simulink model "Modell_PID"  (R2023a)
settings: Solver=VariableStepAuto  StartTime=0.0  StopTime=480  FixedStep=1/30  RelTol=1e-3
undefined symbols (not defined in the file or in its folder): DiscIntNeverNeededParam, dsys, gray, LF, none, videoinput
libraries: instrumentseriallib x3, visiontextngfix x2, slident x2, svdutilitieslib x1, imaqlib x1, simulink_extras x1, simulink x1
settings Model: Creator=Legenden-PC  LastModifiedBy=Legenden-PC
settings OptimizationCC: ReuseModelBlockBuffer=off

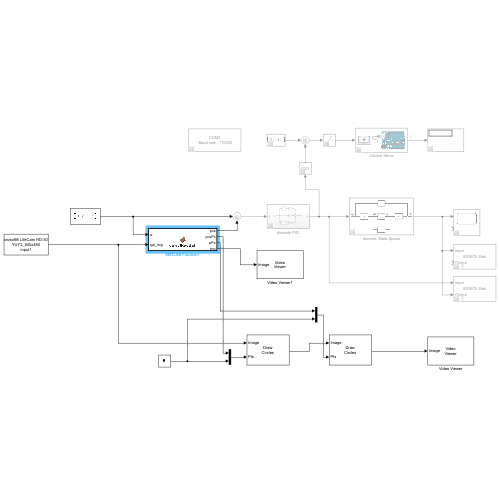
[thumbnail: Simulink's stored preview of the top-level diagram]
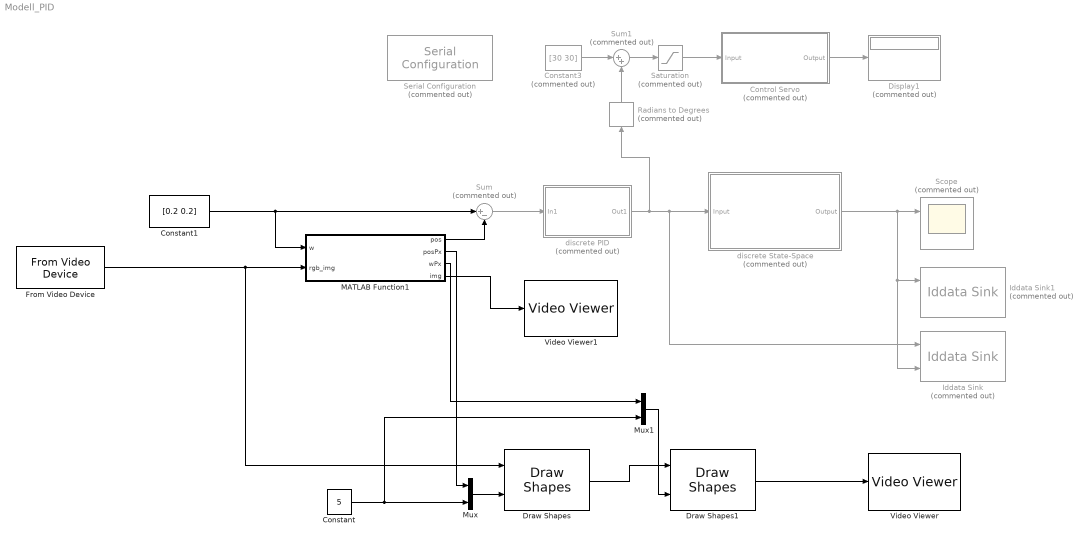
== system Modell_PID ==
  Constant : Constant  Value=5  VectorParams1D=off
  Constant1 : Constant  Value=[0.2 0.2]  SampleTime=1/30
  Constant3 : Constant  Commented=on  Value=[30 30]
  Control Servo : Subsystem  Commented=on
      mask Display: image('C:\Users\Legenden-PC\Desktop\arduino_usb.png'); % Use "Edit Image" on toolstrip to change.
  Display1 : Display  Commented=on
  Draw Shapes : visiontextngfix/Draw Shapes  shape=Circles  fill=off  lineWidth=3  fillClrSource=Specify via dialog  display=Black  intensity=200  color=[200 255 100]  opacity=0.6  viewport=Entire image  antialiasing=off  inType=Obsolete  imagePorts=One multidimensional signal  roundingMode=Floor  overflowMode=off  memoryMode=Specify word length  memoryWordLength=16  prodOutputMode=Binary point scaling  prodOutputWordLength=32  prodOutputFracLength=14  memoryFracLength=15
  Draw Shapes1 : visiontextngfix/Draw Shapes  shape=Circles  fill=off  lineWidth=3  fillClrSource=Specify via dialog  display=Black  intensity=200  color=[200 255 100]  opacity=0.6  viewport=Entire image  antialiasing=off  inType=Obsolete  imagePorts=One multidimensional signal  roundingMode=Floor  overflowMode=off  memoryMode=Specify word length  memoryWordLength=16  prodOutputMode=Binary point scaling  prodOutputWordLength=32  prodOutputFracLength=14  memoryFracLength=15
  From Video Device : imaqlib/From Video Device  DeviceMenu=winvideo 2 (Microsoft® LifeCam HD-3000)  Device=winvideo 2 (Microsoft® LifeCam HD-3000)  ObjConstructor=videoinput('winvideo', 2)  VideoFormatMenu=YUY2_640x480  VideoFormat=YUY2_640x480  VideoSource=input1  ROIPosition=[0 60 480 480]  EnableHWTrigger=off  TriggerConfiguration=none/none  SampleTime=1/30  OutputPortsMode=One multidimensional signal  DataType=single  CanDoHWTrigger=no  ReturnedColorSpace=rgb  BlockHandle=10250.0001  ROIWidth=480  ROIHeight=480  ROIColumn=60  ROIRow=0  EngXMLPath=C:\Program Files\MATLAB\R2023a\toolbox\imaq\imaq\private  DevXMLPath=C:\ProgramData\MATLAB\SupportPackages\R2023a\toolbox\imaq\supportpackages\genericvideo\adaptor\win64  EngLibPath=C:\Program Files\MATLAB\R2023a\toolbox\imaq\imaqblks\imaqmex\win64  ColorSpace=rgb  BayerSensorAlignment=grbg  ImaqMode=off
  Iddata Sink : slident/Iddata Sink  Commented=on  datasetname=ymodel  Ts=1/30  isu=off  isy=off
  Iddata Sink1 : slident/Iddata Sink  Commented=on  datasetname=w_vs_model  Ts=1/30  isu=off  isy=off
  MATLAB Function1 : MATLAB Function  TreatAsAtomicUnit=on
  Mux : Mux  Inputs=2
  Mux1 : Mux  Inputs=2
  Radians to Degrees : simulink_extras/Transformations/Radians to Degrees  Commented=on
  Saturation : Saturate  Commented=on  UpperLimit=60  LowerLimit=0
  Scope : Scope  Commented=on  NumInputPorts=2
  Serial Configuration : instrumentseriallib/Serial Configuration  Priority=-200000  Commented=on  PortSel=COM3  Port=COM3  ComPort=COM3  BaudRate=115200  DataBits=8  Parity=none  StopBits=1  ByteOrder=little-endian  FlowControl=none  Timeout=10  SimulateUsing=Interpreted execution  BlockInModel=on  aMode=1
  Sum : Sum  Commented=on  Inputs=|+-
  Sum1 : Sum  Commented=on  Inputs=|++
  Video Viewer : VideoViewer  colormapValue=gray(256)  FigPos=[1 1030 1920 930]
  Video Viewer1 : VideoViewer  FigPos=[470 761 614 489]
  discrete PID : Subsystem  Commented=on
  discrete State-Space : Subsystem  Commented=on
      mask Display: image('$imagefile'); % Use "Edit Image" on toolstrip to change.
  wires:
  discrete State-Space/1(Output) -> Iddata Sink1/1, Iddata Sink/2, Scope/1
  Sum/1 -> discrete PID/1(In1)
  discrete PID/1(Out1) -> Iddata Sink/1, discrete State-Space/1(Input), Radians to Degrees/1
  From Video Device/1 -> Draw Shapes/1, MATLAB Function1/2(rgb_img)
  Mux/1 -> Draw Shapes/2
  Constant/1 -> Mux1/2, Mux/2
  MATLAB Function1/2(posPx) -> Mux/1
  MATLAB Function1/1(pos) -> Sum/2
  Saturation/1 -> Control Servo/1(Input)
  Sum1/1 -> Saturation/1
  Control Servo/1(Output) -> Display1/1
  Radians to Degrees/1 -> Sum1/2
  Constant3/1 -> Sum1/1
  Draw Shapes/1 -> Draw Shapes1/1
  Draw Shapes1/1 -> Video Viewer/1
  Mux1/1 -> Draw Shapes1/2
  MATLAB Function1/3(wPx) -> Mux1/1
  Constant1/1 -> Sum/1, MATLAB Function1/1(w)
  MATLAB Function1/4(img) -> Video Viewer1/1

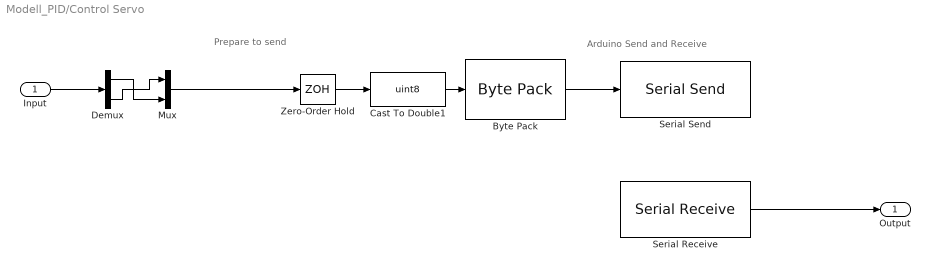
== system Modell_PID/Control Servo ==
  note: Prepare to send
  note: Arduino Send and Receive
  Input : Inport
  Byte Pack : svdutilitieslib/Byte Pack  maskPackedDataType=uint8  datatypes={'uint8'}  byteAlign=2  blockPlatform=arduinoert
  Cast To Double1 : DataTypeConversion  OutDataTypeStr=uint8  SaturateOnIntegerOverflow=off  RndMeth=Floor
  Demux : Demux  Outputs=2
  Mux : Mux  Inputs=2
  Serial Receive : instrumentseriallib/Serial Receive  PortSel=COM3  Port=COM3  ComPort=COM3  DataType=uint8  SaveDataType=uint8  ToggleHeader=on  Header=[ 65 ]  ToggleTerminator=on  Terminator=LF ('\n')  CustomTerminator=[]  InputFormat=Column major  ToggleDataSize=on  DataSize="[1  2]"  EnableBlockingMode=on  ActionDataUnavailable=Output last received value  ActionWhenDataUnavailable=Output last received value  CustomValue=0  SampleTime=0.01  SimulateUsing=Interpreted execution  BlockInModel=on  aMode=1
  Serial Send : instrumentseriallib/Serial Send  PortSel=COM3  Port=COM3  ComPort=COM3  Header=[]  Terminator=<none>  CustomTerminator=[]  EnableBlockingMode=on  SimulateUsing=Interpreted execution  BlockInModel=on  aMode=1
  Zero-Order Hold : ZeroOrderHold  SampleTime=0.01
  Output : Outport
  wires:
  Cast To Double1/1 -> Byte Pack/1
  Byte Pack/1 -> Serial Send/1
  Serial Receive/1 -> Output/1
  Zero-Order Hold/1 -> Cast To Double1/1
  Input/1 -> Demux/1
  Demux/1 -> Mux/2
  Demux/2 -> Mux/1
  Mux/1 -> Zero-Order Hold/1

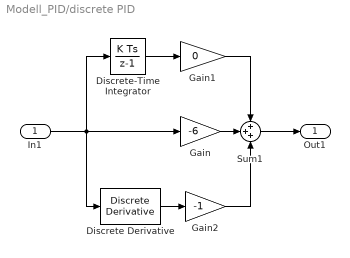
== system Modell_PID/discrete PID ==
  In1 : Inport
  Discrete Derivative : simulink/Discrete/Discrete Derivative  gainval=1.0  ICPrevScaledInput=0.0  OutMin=[]  OutMax=[]  OutDataType=fixdt(1, 16)  OutScaling=2^-10  DoSatur=off
  Discrete-Time Integrator : DiscreteIntegrator  SampleTime=1/30  ICPrevOutput=DiscIntNeverNeededParam  ICPrevScaledInput=DiscIntNeverNeededParam
  Gain : Gain  Gain=-6
  Gain1 : Gain  Gain=0
  Gain2 : Gain  Gain=-1
  Sum1 : Sum  Inputs=+++
  Out1 : Outport
  wires:
  Gain/1 -> Sum1/2
  Gain2/1 -> Sum1/3
  Discrete Derivative/1 -> Gain2/1
  In1/1 -> Discrete Derivative/1, Discrete-Time Integrator/1, Gain/1
  Discrete-Time Integrator/1 -> Gain1/1
  Gain1/1 -> Sum1/1
  Sum1/1 -> Out1/1

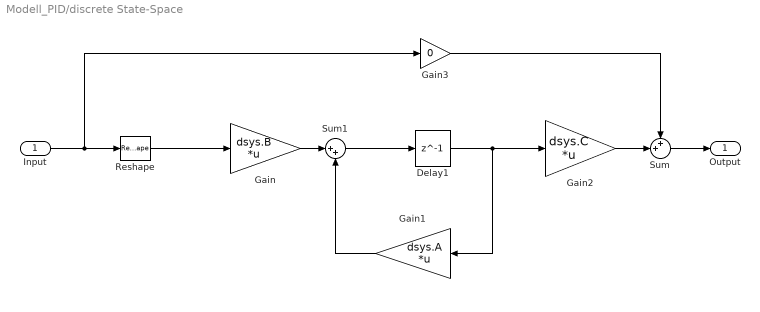
== system Modell_PID/discrete State-Space ==
  Input : Inport
  Delay1 : Delay  DelayLength=1  InitialCondition=[0.2 0 0.2 0]'
  Gain : Gain  Gain=dsys.B  Multiplication=Matrix(K*u)
  Gain1 : Gain  Gain=dsys.A  Multiplication=Matrix(K*u)
  Gain2 : Gain  Gain=dsys.C  Multiplication=Matrix(K*u)
  Gain3 : Gain  Gain=0
  Reshape : Reshape
  Sum : Sum  Inputs=++|
  Sum1 : Sum  Inputs=|++
  Output : Outport
  wires:
  Input/1 -> Reshape/1, Gain3/1
  Gain/1 -> Sum1/1
  Sum1/1 -> Delay1/1
  Delay1/1 -> Gain1/1, Gain2/1
  Gain1/1 -> Sum1/2
  Gain2/1 -> Sum/2
  Gain3/1 -> Sum/1
  Sum/1 -> Output/1
  Reshape/1 -> Gain/1

== matlab function Modell_PID/MATLAB Function1 ==
  data: w input; pos output; rgb_img input; posPx output; wPx output; img output
function [pos,posPx,wPx,img] = detectRedBall(w,rgb_img)
    persistent hBlob Px2m
    
    if isempty(hBlob)
        hBlob = vision.BlobAnalysis("AreaOutputPort",1, ...
                                    "ExcludeBorderBlobs",0, ...
                                    "MinimumBlobArea",1000, ...
                                    "MaximumBlobArea",5000);
        Px2m = [0.4/480 0.4/480];
    end

    bw = im2gray(rgb_img)>=170/255; %rgb_img(:,:,1) >= 99/255 & rgb_img(:,:,2) <= 50/255 & rgb_img(:,:,3) <= 50/255;
    [area, bbox, detectBall] = hBlob(bw);


    [va,idx] = max(area);

    if va
        posPx = double(detectBall(idx(1,1),1:2));
        wPx = (w);%*1./Px2m);
        pos = double(posPx(idx(1,1),1:2)).*Px2m;
    else
        posPx = double([0 0]);
        wPx = (w);%*1./Px2m);
        pos = w';
    end

    img = bw;
end
